simulink model "Lab02"  (R2018a)
settings: Solver=VariableStepAuto  StartTime=0  StopTime=10  RelTol=1e-3
undefined symbols (not defined in the file or in its folder): K
settings Model: Creator=rodrigue  LastModifiedBy=rodrigue
settings CodeAppCC: StateflowObjectComments=on

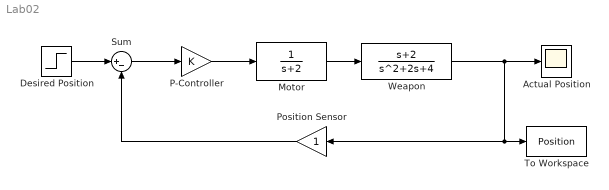
== system Lab02 ==
  Actual Position : Scope
  Desired Position : Step  SampleTime=0
  Motor : TransferFcn  Numerator=1  Denominator=[1 2]
  P-Controller : Gain  Gain=K
  Position Sensor : Gain
  Sum : Sum  Inputs=|+-
  To Workspace : ToWorkspace  VariableName=Position  SampleTime=-1
  Weapon : TransferFcn  Numerator=[1, 2]  Denominator=[1, 2, 4]
  wires:
  Motor/1 -> Weapon/1
  Weapon/1 -> Position Sensor/1, To Workspace/1, Actual Position/1
  P-Controller/1 -> Motor/1
  Desired Position/1 -> Sum/1
  Sum/1 -> P-Controller/1
  Position Sensor/1 -> Sum/2
